simulink model "G8_Test"  (R2021a)
settings: Solver=VariableStepAuto  StartTime=0.0  StopTime=inf  RelTol=1e-3
undefined symbols (not defined in the file or in its folder): DiscIntNeverNeededParam
libraries: simulink x4, instrumentlib x2, dspstat3 x1, dspindex x1, realtime_pacer_lib x1, pid_lib x1, SignalEditorBlockLib x1
settings Model: Creator=errikos  LastModifiedBy=AERO-REMOTELABS
settings SolverCC: AlgebraicLoopSolver=TrustRegion
settings DataIOCC: ReturnWorkspaceOutputs=off
settings DebuggingCC: SFMachineParentedDataDiag=warning  ArithmeticOperatorsInVariantConditions=warning
settings SFSimCC: CustomCodeUndefinedFunction=UseInterfaceOnly

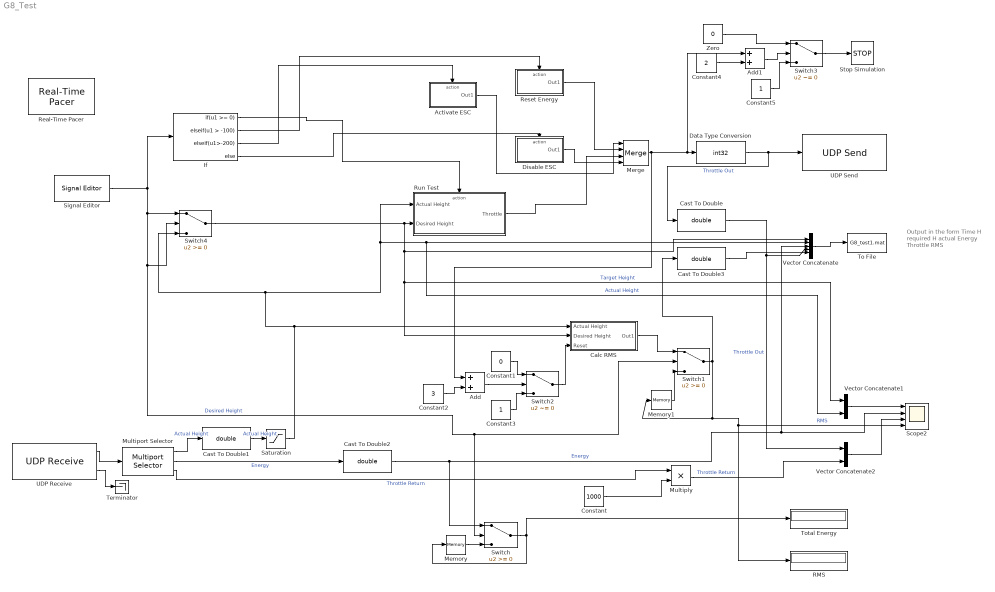
== system G8_Test ==
  note: Output in the form
      | Time
      | H required
      | H actual
      | Energy
      | Throttle
      | RMS
  Activate ESC : Subsystem  TreatAsAtomicUnit=on
  Add : Sum
  Add1 : Sum
  Calc RMS : Subsystem
  Cast To Double{,1..3} (4 alike) : DataTypeConversion  OutDataTypeStr=double
  Constant : Constant  Value=1000
  Constant1 : Constant  Value=0
  Constant2 : Constant  Value=3
  Constant3 : Constant
  Constant4 : Constant  Value=2
  Constant5 : Constant
  Data Type Conversion : DataTypeConversion  OutDataTypeStr=int32
  Disable ESC : Subsystem  TreatAsAtomicUnit=on
  If : If  IfExpression=u1 >= 0  ElseIfExpressions=u1 > -100 , u1>-200
  Memory : Memory
  Memory1 : Memory
  Merge : Merge  Inputs=4
  Multiply : Product
  Multiport Selector : dspindex/Multiport Selector  rowsOrCols=Columns  idxCellArray={ 1, 2,3}  idxErrMode=Clip and Warn
  RMS : Display
  Real-Time Pacer : realtime_pacer_lib/Real-Time Pacer  simTimePerRealTime=1
  Reset Energy : Subsystem  TreatAsAtomicUnit=on
  Run Test : Subsystem  TreatAsAtomicUnit=on
  Saturation : Saturate  UpperLimit=1.7  LowerLimit=0
  Scope2 : Scope  NumInputPorts=4
  Signal Editor : SignalEditorBlockLib/Signal Editor  FileName=testmission2021.mat  ActiveScenario=Scenario  ActiveSignal=Signal 1  IsBus=off  OutputBusObjectStr=Bus: BusObject  SampleTime=0.05  ZeroCross=off  OutputAfterFinalValue=Setting to zero  Unit=inherit  PreserveSignalName=on
  Stop Simulation : Stop
  Switch : Switch
  Switch1 : Switch
  Switch2 : Switch  Criteria=u2 ~= 0
  Switch3 : Switch  Criteria=u2 ~= 0  ZeroCross=off
  Switch4 : Switch
  Terminator : Terminator
  To File : ToFile  Filename=G8_test1.mat
  Total Energy : Display
  UDP Receive : instrumentlib/UDP Receive  Host=192.168.0.110  Port=4000  LocalPort=8888  EnablePortSharing=on  GetLatestData=on  DataSize="[1  3]"  DataType=single  ASCIIFormatting=%f%f  Terminator=LF  ByteOrder=LittleEndian  EnableBlockingMode=off  Timeout=10  SampleTime=0.05  LocalAddress=192.168.0.100
  UDP Send : instrumentlib/UDP Send  Host=192.168.0.110  Port=4000  LocalPort=-1  EnablePortSharing=on  ByteOrder=LittleEndian  OutputDatagramPacketSize=4  EnableBlockingMode=on  LocalAddress=192.168.0.100
  Vector Concatenate : Concatenate  NumInputs=5
  Vector Concatenate1 : Concatenate
  Vector Concatenate2 : Concatenate
  Zero : Constant  Value=0  OutDataTypeStr=Inherit: Inherit via back propagation
  wires:
  UDP Receive/1 -> Multiport Selector/1
  Multiport Selector/1 -> Cast To Double1/1  "Actual Height"
  Multiport Selector/2 -> Cast To Double2/1  "Energy"
  Run Test/1("Throttle ") -> Merge/3
  Data Type Conversion/1 -> Cast To Double/1, UDP Send/1  "Throttle Out"
  Multiport Selector/3 -> Multiply/1  "Throttle Return"
  Multiply/1 -> Vector Concatenate2/2  "Throttle Return"
  Constant/1 -> Multiply/2
  Signal Editor/1 -> Switch4/2, Switch1/2, Switch/2, Switch4/1, If/1  "Desired Height"
  Merge/1 -> Add/1, Add1/1, Data Type Conversion/1
  Vector Concatenate/1 -> To File/1
  If/1 -> Run Test/Action
  If/2 -> Reset Energy/Action
  If/3 -> Activate ESC/Action
  If/4 -> Disable ESC/Action
  Activate ESC/1(Out1) -> Merge/1
  Disable ESC/1(Out1) -> Merge/4
  Switch/1 -> Memory/1, Total Energy/1
  Cast To Double/1 -> Vector Concatenate2/1, Vector Concatenate/4  "Throttle Out"
  Saturation/1 -> Switch4/3, Run Test/1(Actual Height), Vector Concatenate1/2, Vector Concatenate/2, Calc RMS/1(Actual Height)  "Actual Height"
  Cast To Double2/1 -> Switch/1, Scope2/2, Vector Concatenate/3  "Energy"
  Cast To Double3/1 -> Vector Concatenate/5
  Memory/1 -> Switch/3
  Switch1/1 -> RMS/1, Scope2/4, Memory1/1, Cast To Double3/1  "RMS"
  Memory1/1 -> Switch1/3
  Calc RMS/1(Out1) -> Switch1/1
  Switch2/1 -> Calc RMS/3(Reset)
  Constant1/1 -> Switch2/1
  Constant2/1 -> Add/2
  Add/1 -> Switch2/2
  Constant3/1 -> Switch2/3
  Reset Energy/1(Out1) -> Merge/2
  Switch3/1 -> Stop Simulation/1
  Zero/1 -> Switch3/1
  Add1/1 -> Switch3/2
  Constant4/1 -> Add1/2
  Constant5/1 -> Switch3/3
  Vector Concatenate2/1 -> Scope2/3
  Vector Concatenate1/1 -> Scope2/1
  Switch4/1 -> Vector Concatenate/1, Vector Concatenate1/1, Calc RMS/2(Desired Height), Run Test/2(Desired Height)  "Target Height"
  Cast To Double1/1 -> Saturation/1  "Actual Height"
  UDP Receive/2 -> Terminator/1

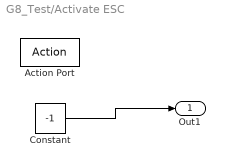
== system G8_Test/Activate ESC ==
  Action Port : ActionPort  ActionPortLabel=elseif( u1>-200)
  Constant : Constant  Value=-1  SampleTime=0.05
  Out1 : Outport  VectorParamsAs1DForOutWhenUnconnected=off
  wires:
  Constant/1 -> Out1/1

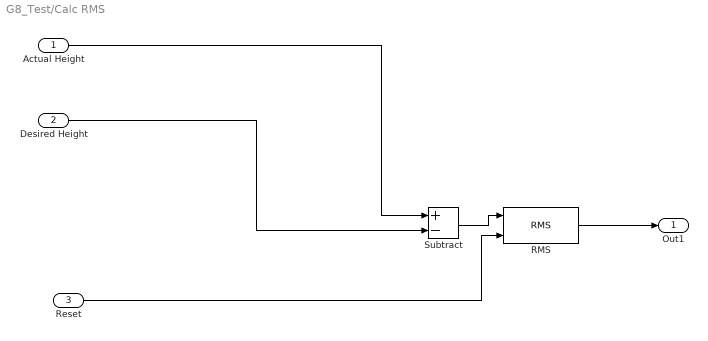
== system G8_Test/Calc RMS ==
  Actual Height : Inport
  Desired Height : Inport  Port=2
  Reset : Inport  Port=3
  RMS : dspstat3/RMS  run=on  directionMode=Each column  dimension=1  reset_popup=Non-zero sample
  Subtract : Sum  Inputs=+-
  Out1 : Outport  VectorParamsAs1DForOutWhenUnconnected=off
  wires:
  Desired Height/1 -> Subtract/2
  Actual Height/1 -> Subtract/1
  RMS/1 -> Out1/1
  Subtract/1 -> RMS/1
  Reset/1 -> RMS/2

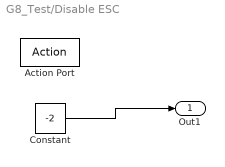
== system G8_Test/Disable ESC ==
  Action Port : ActionPort  ActionPortLabel=else
  Constant : Constant  Value=-2  SampleTime=0.05
  Out1 : Outport  VectorParamsAs1DForOutWhenUnconnected=off
  wires:
  Constant/1 -> Out1/1

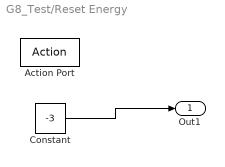
== system G8_Test/Reset Energy ==
  Action Port : ActionPort  ActionPortLabel=elseif(u1 > -100 )
  Constant : Constant  Value=-3  SampleTime=0.05
  Out1 : Outport  VectorParamsAs1DForOutWhenUnconnected=off
  wires:
  Constant/1 -> Out1/1

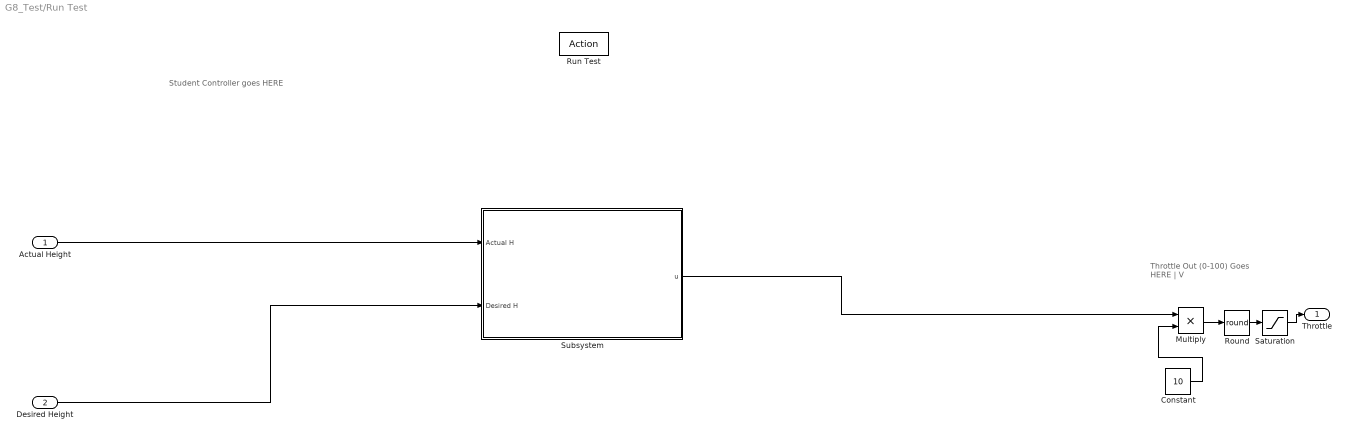
== system G8_Test/Run Test ==
  note: Throttle Out (0-100)
      | Goes HERE
      |            |
      | 	   V
  note: Student Controller goes HERE
  Actual Height : Inport
  Desired Height : Inport  Port=2
  Run Test : ActionPort  ActionPortLabel=if(u1 >= 0)
  Constant : Constant  Value=10
  Multiply : Product
  Round : Rounding  Operator=round
  Saturation : Saturate  UpperLimit=1000  LowerLimit=0
  Subsystem : Subsystem
  "Throttle " : Outport  VectorParamsAs1DForOutWhenUnconnected=off
  wires:
  Saturation/1 -> "Throttle "/1
  Constant/1 -> Multiply/2
  Multiply/1 -> Round/1
  Round/1 -> Saturation/1
  Subsystem/1(u) -> Multiply/1
  Actual Height/1 -> Subsystem/1(Actual H)
  Desired Height/1 -> Subsystem/2(Desired H)

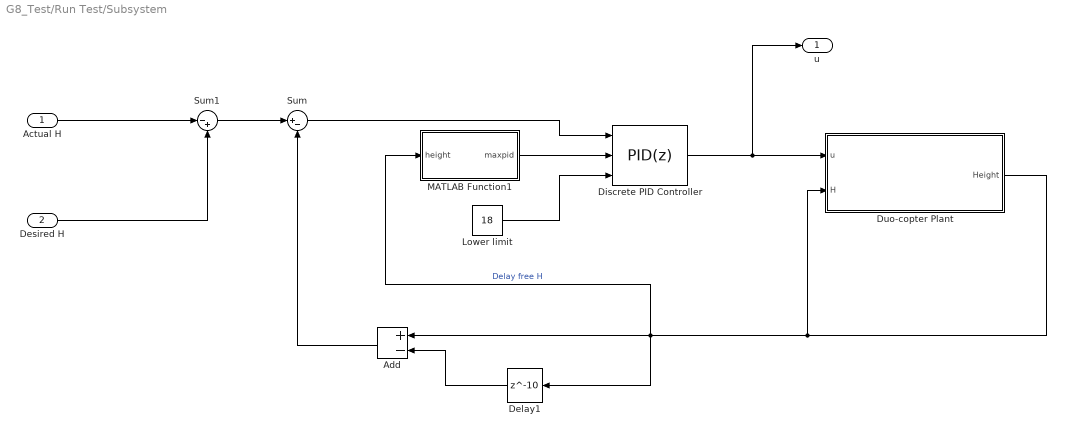
== system G8_Test/Run Test/Subsystem ==
  Actual H : Inport
  Desired H : Inport  Port=2
  Add : Sum  Inputs=+-
  Delay1 : Delay  DelayLength=10  InitialCondition=0  SampleTime=0.05
  Discrete PID Controller : pid_lib/PID Controller  Controller=PID  Form=Parallel  TimeDomain=Discrete-time  UseExternalTs=off  SampleTime=0.05  IntegratorMethod=Forward Euler  FilterMethod=Forward Euler  ControllerParametersSource=internal  P=18  I=16  D=13  UseFilter=off  N=70  TunerSelectOption=Transfer Function Based (PID Tuner App)  InitialConditionSource=internal  InitialConditionForIntegrator=0  InitialConditionForFilter=0  DifferentiatorICPrevScaledInput=0  ExternalReset=none  TrackingMode=off  Kt=1  LimitOutput=on  SatLimitsSource=external  UpperSaturationLimit=50  LowerSaturationLimit=0  LinearizeAsGain=off  AntiWindupMode=back-calculation  Kb=1  POutMin=[]  POutMax=[]  IOutMin=[]  IOutMax=[]  DOutMin=[]  DOutMax=[]  NOutMin=[]  NOutMax=[]  SumOutMin=[]  SumOutMax=[]  SaturationOutMin=[]  SaturationOutMax=[]  PParamMin=[]  PParamMax=[]  IParamMin=[]  IParamMax=[]  DParamMin=[]  DParamMax=[]  NParamMin=[]  NParamMax=[]  KbParamMin=[]  KbParamMax=[]  KtParamMin=[]  KtParamMax=[]  KbOutMin=[]  KbOutMax=[]  KtOutMin=[]  KtOutMax=[]  IntegratorOutMin=[]  IntegratorOutMax=[]  FilterOutMin=[]  FilterOutMax=[]  SumI1OutMin=[]  SumI1OutMax=[]  SumI2OutMin=[]  SumI2OutMax=[]  SumI3OutMin=[]  SumI3OutMax=[]  SumI4OutMin=[]  SumI4OutMax=[]  SumDOutMin=[]  SumDOutMax=[]  DifferentiatorOutMin=[]  DifferentiatorOutMax=[]  FilterDiffOutCoefMin=[]  FilterDiffOutCoefMax=[]  ReciprocalOutMin=[]  ReciprocalOutMax=[]  SumDenOutMin=[]  SumDenOutMax=[]  SumNumOutMin=[]  SumNumOutMax=[]  DivideOutMin=[]  DivideOutMax=[]  UdiffTsProdOutMin=[]  UdiffTsProdOutMax=[]  NTsProdOutMin=[]  NTsProdOutMax=[]  UintegralTsProdOutMin=[]  UintegralTsProdOutMax=[]  UngainTsProdOutMin=[]  UngainTsProdOutMax=[]  IntegratorContinuousStateAttributes=''  IntegratorStateMustResolveToSignalObject=off  IntegratorRTWStateStorageClass=Auto  FilterContinuousStateAttributes=''  FilterStateMustResolveToSignalObject=off  FilterRTWStateStorageClass=Auto  ParallelPVariant=InternalParameters  IdealPVariant=Disabled  IVariant=InternalParameters  DVariant=InternalParameters  IntegratorVariant=Discrete  SatVariant=External  AWVariant=BackCalculation  PCopyVariant=Disabled  TRVariant=Disabled  FdbkBlocksVariant=Forward  IdealPFdbkVariant=Disabled  SatFdbkVariant=Disabled  DerivativeFilterVariant=Differentiator  NVariant=Passthrough  NCopyVariant=Disabled_SignalSpec  FilterICVariant=InternalICsDifferentiator  IntegratorICVariant=InternalICs  ExternalResetVariant=Disabled  TRSumVariant=Passthrough  SumFdbkVariant=Disabled  SumVariant=Sum_PID  TsampFilterVariant=InternalTs  TsampNgainVariant=Passthrough  TsampIntegralVariant=Passthrough  ExternalSaturationOutDataTypeStr=Inherit: Same as second input
  Duo-copter Plant : Subsystem
  Lower limit : Constant  Value=18  SampleTime=0.05
  MATLAB Function1 : MATLAB Function  TreatAsAtomicUnit=on
  Sum : Sum  Inputs=|+-
  Sum1 : Sum  Inputs=|-+
  u : Outport
  wires:
  Lower limit/1 -> Discrete PID Controller/3
  Add/1 -> Sum/2
  Duo-copter Plant/1(Height) -> Duo-copter Plant/2(H), Delay1/1, Add/1, MATLAB Function1/1(height)  "Delay free H"
  Delay1/1 -> Add/2
  MATLAB Function1/1(maxpid) -> Discrete PID Controller/2
  Sum/1 -> Discrete PID Controller/1
  Desired H/1 -> Sum1/2
  Sum1/1 -> Sum/1
  Discrete PID Controller/1 -> Duo-copter Plant/1(u), u/1
  Actual H/1 -> Sum1/1

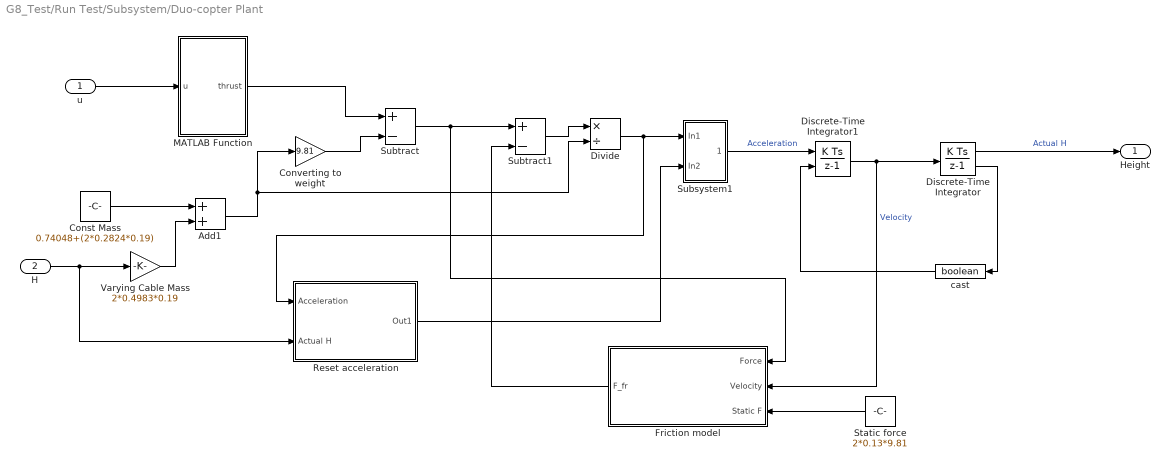
== system G8_Test/Run Test/Subsystem/Duo-copter Plant ==
  u : Inport
  H : Inport  Port=2
  " Converting to weight" : Gain  Gain=9.81
  Add1 : Sum
  Const Mass : Constant  Value=0.74048+(2*0.2824*0.19)  SampleTime=0.05
  Discrete-Time Integrator : DiscreteIntegrator  SampleTime=0.05  LimitOutput=on  UpperSaturationLimit=1.44  LowerSaturationLimit=0  ShowSaturationPort=on  ICPrevOutput=DiscIntNeverNeededParam  ICPrevScaledInput=DiscIntNeverNeededParam
  Discrete-Time Integrator1 : DiscreteIntegrator  ExternalReset=rising  SampleTime=0.05  UpperSaturationLimit=0.2  LowerSaturationLimit=-0.8  ICPrevOutput=DiscIntNeverNeededParam  ICPrevScaledInput=DiscIntNeverNeededParam
  Divide : Product  Inputs=*/
  Friction model : Subsystem
  MATLAB Function : MATLAB Function  TreatAsAtomicUnit=on
  Reset acceleration : Subsystem
  Static force : Constant  Value=2*0.13*9.81  SampleTime=0.05
  Subsystem1 : Subsystem
  Subtract : Sum  Inputs=+-
  Subtract1 : Sum  Inputs=+-
  Varying Cable Mass : Gain  Gain=2*0.4983*0.19
  cast : DataTypeConversion  OutDataTypeStr=boolean  SaturateOnIntegerOverflow=on  RndMeth=Zero
  Height : Outport
  wires:
  H/1 -> Reset acceleration/2(Actual H), Varying Cable Mass/1
  Reset acceleration/1(Out1) -> Subsystem1/2(In2)
  Discrete-Time Integrator/2 -> cast/1
  Subsystem1/1("  ") -> Discrete-Time Integrator1/1  "Acceleration"
  Const Mass/1 -> Add1/1
  Add1/1 -> " Converting to weight"/1, Divide/2
  Friction model/1(F_fr) -> Subtract1/2
  Static force/1 -> Friction model/3(Static F)
  Discrete-Time Integrator/1 -> Height/1  "Actual H"
  Discrete-Time Integrator1/1 -> Friction model/2(Velocity), Discrete-Time Integrator/1  "Velocity"
  Divide/1 -> Reset acceleration/1(Acceleration), Subsystem1/1(In1)
  cast/1 -> Discrete-Time Integrator1/2
  Varying Cable Mass/1 -> Add1/2
  Subtract1/1 -> Divide/1
  Subtract/1 -> Subtract1/1, Friction model/1(Force)
  " Converting to weight"/1 -> Subtract/2
  u/1 -> MATLAB Function/1(u)
  MATLAB Function/1(thrust) -> Subtract/1

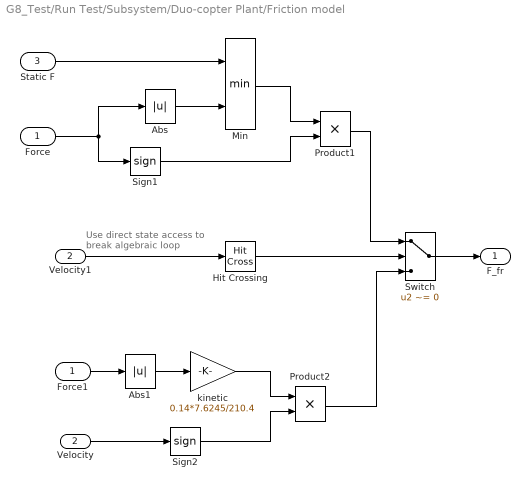
== system G8_Test/Run Test/Subsystem/Duo-copter Plant/Friction model ==
  note: Use direct state access to
      | break algebraic loop
  Force : Inport  SampleTime=0.05
  Velocity : Inport  Port=2
  Static F : Inport  Port=3  SampleTime=0.05
  Abs : Abs  SaturateOnIntegerOverflow=on
  Abs1 : Abs  SaturateOnIntegerOverflow=on
  Force1 : InportShadow  SampleTime=0.05
  Hit Crossing : HitCross
  Min : MinMax  Inputs=2  InputSameDT=on  SaturateOnIntegerOverflow=on
  Product1 : Product  InputSameDT=on  SaturateOnIntegerOverflow=on  OutDataTypeStr=Inherit: Same as first input
  Product2 : Product  InputSameDT=on  SaturateOnIntegerOverflow=on  OutDataTypeStr=Inherit: Same as first input
  Sign1 : Signum
  Sign2 : Signum
  Switch : Switch  Criteria=u2 ~= 0  Threshold=0.5  InputSameDT=on
  Velocity1 : InportShadow  Port=2
  kinetic : Gain  Gain=0.14*7.6245/210.4
  F_fr : Outport  InitialOutput=0  VectorParamsAs1DForOutWhenUnconnected=off
  wires:
  Product1/1 -> Switch/1
  Sign1/1 -> Product1/2
  Hit Crossing/1 -> Switch/2
  Force/1 -> Abs/1, Sign1/1
  Velocity/1 -> Sign2/1
  Switch/1 -> F_fr/1
  Min/1 -> Product1/1
  Abs/1 -> Min/2
  Static F/1 -> Min/1
  Product2/1 -> Switch/3
  Velocity1/1 -> Hit Crossing/1
  Sign2/1 -> Product2/2
  kinetic/1 -> Product2/1
  Force1/1 -> Abs1/1
  Abs1/1 -> kinetic/1

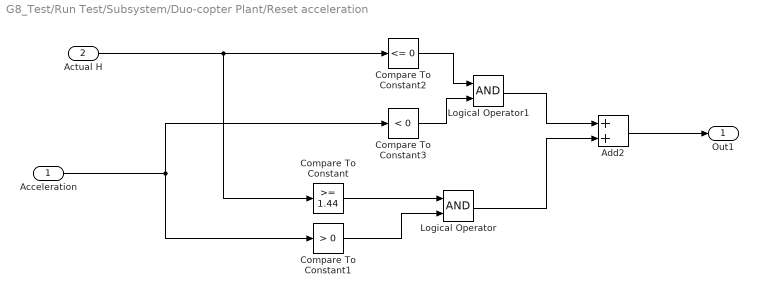
== system G8_Test/Run Test/Subsystem/Duo-copter Plant/Reset acceleration ==
  Acceleration : Inport
  Actual H : Inport  Port=2
  Add2 : Sum
  Compare To Constant : simulink/Logic and Bit Operations/Compare To Constant  relop=>=  const=1.44  OutDataTypeStr=boolean
  Compare To Constant1 : simulink/Logic and Bit Operations/Compare To Constant  relop=>  const=0  OutDataTypeStr=boolean
  Compare To Constant2 : simulink/Logic and Bit Operations/Compare To Constant  relop=<=  const=0  OutDataTypeStr=boolean
  Compare To Constant3 : simulink/Logic and Bit Operations/Compare To Constant  relop=<  const=0  OutDataTypeStr=boolean
  Logical Operator : Logic  AllPortsSameDT=off  OutDataTypeStr=boolean
  Logical Operator1 : Logic  AllPortsSameDT=off  OutDataTypeStr=boolean
  Out1 : Outport
  wires:
  Compare To Constant/1 -> Logical Operator/1
  Compare To Constant1/1 -> Logical Operator/2
  Logical Operator/1 -> Add2/2
  Logical Operator1/1 -> Add2/1
  Compare To Constant3/1 -> Logical Operator1/2
  Acceleration/1 -> Compare To Constant3/1, Compare To Constant1/1
  Compare To Constant2/1 -> Logical Operator1/1
  Add2/1 -> Out1/1
  Actual H/1 -> Compare To Constant/1, Compare To Constant2/1

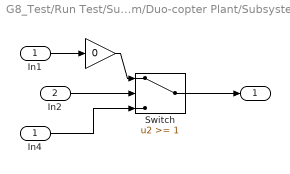
== system G8_Test/Run Test/Subsystem/Duo-copter Plant/Subsystem1 ==
  In1 : Inport  SampleTime=0.05
  In2 : Inport  Port=2  SampleTime=0.05
  " " : Gain  Gain=0
  In4 : InportShadow  SampleTime=0.05
  Switch : Switch  Threshold=1
  "  " : Outport
  wires:
  In1/1 -> " "/1
  In2/1 -> Switch/2
  " "/1 -> Switch/1
  Switch/1 -> "  "/1
  In4/1 -> Switch/3

== matlab function G8_Test/Run Test/Subsystem/Duo-copter Plant/MATLAB Function ==
  data: u input; thrust output
function thrust   = model(u)
%inputs
%       - u:  control vector
%         u(1)- engine throttle as percentage


thrust=2*(-1.406748142176356e-10*u^6+3.062978540873029e-08*u^5-2.097995902290989e-06*u^4+3.239235806681329e-05*u^3+0.001982324981180*u^2+0.021260289345294*u+0.164761238254325);

end

== matlab function G8_Test/Run Test/Subsystem/MATLAB Function1 ==
  data: height input; maxpid output
function maxpid = maxpid(height)

cartmass        = 0.74048;      %kg

cablemass       = 2*(0.4983*0.190*height+0.2824*0.190); %kg

mass = cartmass  + cablemass; %kg

maxt = mass * 9.81 -0.5;

maxpid = 1*(0.000106460047187 * maxt^6 + 0.001682145469029 * maxt^5 - 0.085966748628573 * maxt^4 + 0.915086428052733 * maxt^3 - 4.301170611461207 * maxt^2 + 19.048979026808645 * maxt - 0.819624990299465);
